simulink library "bayesianAscent_cl"  (R2018b)
settings: Solver=VariableStepAuto  StartTime=0.0  StopTime=10.0  RelTol=1e-3
settings Model: Creator=Ayaz  LastModifiedBy=asiddiq2

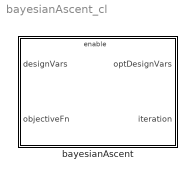
== system bayesianAscent_cl ==
  bayesianAscent : Subsystem  TreatAsAtomicUnit=on  mask{gpTrain=0, gpTrainFval=0, iniOptHyp=0, noiseVars=0, desLims=0, gamma=0, beta=0, iniTauPerc=0, maxIter=0}
      mask prompts: gpTrain "Training desgin set"; gpTrainFval "Training objective function values"; iniOptHyp "Training hyper parameters"; noiseVars "Noise variance"; desLims "Design limits"; iniTauPerc "Initial tau percentage"; maxIter "Max iterations"

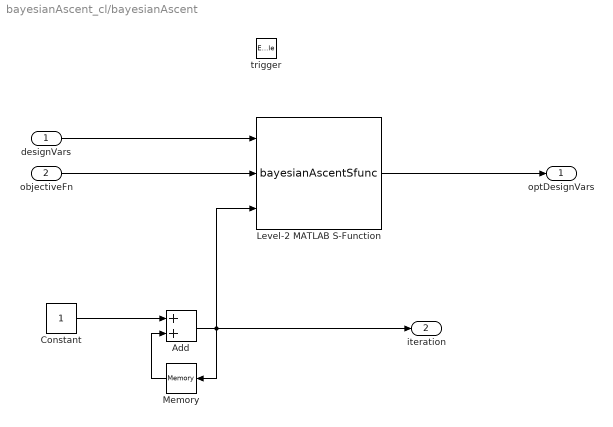
== system bayesianAscent_cl/bayesianAscent ==
  designVars : Inport
  objectiveFn : Inport  Port=2
  trigger : EnablePort
  Add : Sum
  Constant : Constant
  Level-2 MATLAB S-Function : M-S-Function  FunctionName=bayesianAscentSfunc  Parameters=gpTrain,gpTrainFval,iniOptHyp,noiseVars,desLims,gamma,beta,iniTauPerc,maxIter
  Memory : Memory
  optDesignVars : Outport
  iteration : Outport  Port=2
  wires:
  designVars/1 -> Level-2 MATLAB S-Function/1
  objectiveFn/1 -> Level-2 MATLAB S-Function/2
  Level-2 MATLAB S-Function/1 -> optDesignVars/1
  Constant/1 -> Add/1
  Add/1 -> Level-2 MATLAB S-Function/3, Memory/1, iteration/1
  Memory/1 -> Add/2
